simulink model "CtoF"  (R2023b)
settings: Solver=VariableStepAuto  StartTime=0.0  StopTime=10.0  RelTol=1e-3

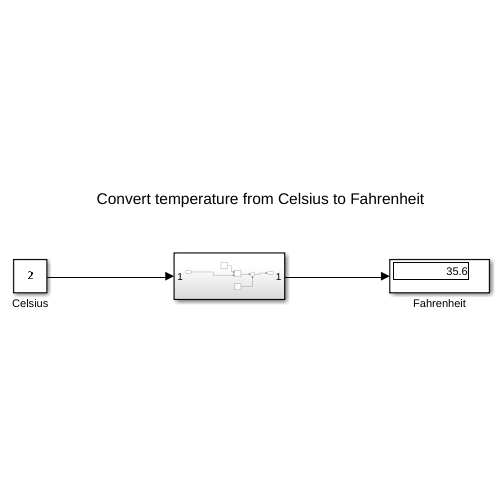
[thumbnail: Simulink's stored preview of the top-level diagram]
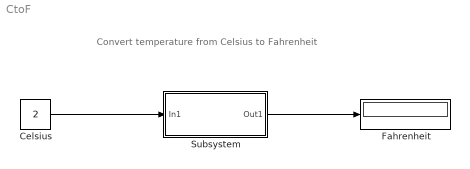
== system CtoF ==
  note: Convert temperature from Celsius to Fahrenheit
  Celsius : Constant  Value=2
  Fahrenheit : Display
  Subsystem : Subsystem
  wires:
  Subsystem/1(Out1) -> Fahrenheit/1
  Celsius/1 -> Subsystem/1(In1)

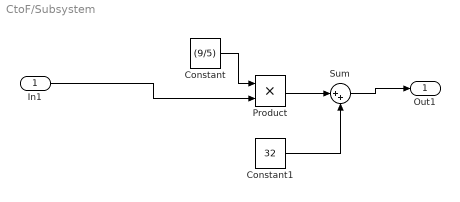
== system CtoF/Subsystem ==
  In1 : Inport
  Constant : Constant  Value=(9/5)
  Constant1 : Constant  Value=32
  Product : Product
  Sum : Sum  Inputs=|++
  Out1 : Outport
  wires:
  In1/1 -> Product/2
  Constant/1 -> Product/1
  Product/1 -> Sum/1
  Constant1/1 -> Sum/2
  Sum/1 -> Out1/1
